simulink model "model_sim_CHBjt7"  (R2023b)
settings: Solver=ode3  StartTime=0.0  StopTime=5  FixedStep=01e-6  RelTol=1e-3
InitFcn:
  | sysinit
StopFcn:
  | code_CHBJT7_stopfcn
values from neighbouring files (symbols this model uses):
  C = 0.0234    [sysinit.m]
  f = 50    [sysinit.m]
  f_switch = 250    [sysinit.m]
  fn = 50    [sysinit.m]
  L = 0.002    [sysinit.m]
  L_1 = eps    [simout_chb_par.m]    (also in simout_chbjt_par.m; sysinit.m)
  L_ori = 0.02    [sysinit.m]
  L_sec = 0.06    [sysinit.m]
  m = 0.95    [sysinit.m]
  P0 = 8e6    (= 8000000)    [sysinit.m]
  R = 1.5    [sysinit.m]
  Source_Amp = 10000    [sysinit.m]
  st = 1e-6    (= 1e-06)    [sysinit.m]
  Td = 15e-7    (= 1.5e-06)    [sysinit.m]
  Ts2 = 0.5e-3    (= 0.0005)    [sysinit.m]
  U_dcN = 2500    [sysinit.m]
  Ul_in = 1900    [sysinit.m]
undefined symbols (not defined in the file or in its folder): magnitude
libraries: spsSeriesRLCBranchLib x120, spsDiodeLib x45, spsIGBTLib x36, spsMeanLib x20, spsCurrentMeasurementLib x15, spsThreePhaseVIMeasurementLib x10, spsOnDelayLib x9, spsMultiWindingTransformerLib x9, spsUniversalBridgeLib x9, simulink x5, spsVoltageMeasurementLib x5, spsRMSLib x4
(part 2 of 3)

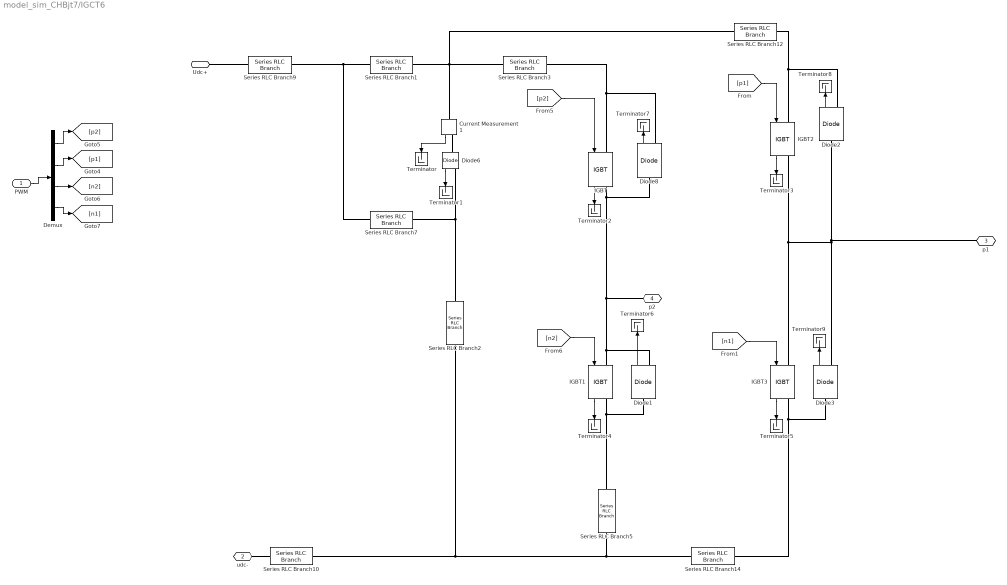
== system model_sim_CHBjt7/IGCT6 ==
  PWM : Inport
  Current Measurement1 : spsCurrentMeasurementLib/Current Measurement  PhasorSimulation=off  OutputType=Complex  PSBequivalent=0
  Demux : Demux
  Diode{1..3,6,8} (5 alike) : spsDiodeLib/Diode  Ron=rto  Lon=0  Vf=vto  IC=0  UseSnubber=off  Rs=500  Cs=250e-9  Measurements=on
  IGBT{,1..3} (4 alike) : spsIGBTLib/IGBT  Ron=rt  Lon=0  Vf=vt  Tf=1e-6  Tt=2e-6  IC=0  Rs=1e5  Cs=inf  Measurements=on
  Series RLC Branch1 : spsSeriesRLCBranchLib/Series RLC Branch  LConnTagsString=__new0  RConnTagsString=__new0  BranchType=RL  Resistance=1e-5  Inductance=3.0E-6  SetiL0=off  InitialCurrent=0  Capacitance=1e-6  Setx0=off  InitialVoltage=0  Measurements=None
  Series RLC Branch10 : spsSeriesRLCBranchLib/Series RLC Branch  LConnTagsString=__new0  RConnTagsString=__new0  BranchType=L  Resistance=1  Inductance=0.4e-6  SetiL0=off  InitialCurrent=0  Capacitance=1e-6  Setx0=off  InitialVoltage=0  Measurements=None
  Series RLC Branch12 : spsSeriesRLCBranchLib/Series RLC Branch  LConnTagsString=__new0  RConnTagsString=__new0  BranchType=RL  Resistance=1e-5  Inductance=1E-9  SetiL0=off  InitialCurrent=0  Capacitance=1e-6  Setx0=off  InitialVoltage=0  Measurements=None
  Series RLC Branch14 : spsSeriesRLCBranchLib/Series RLC Branch  LConnTagsString=__new0  RConnTagsString=__new0  BranchType=L  Resistance=1  Inductance=1E-7  SetiL0=off  InitialCurrent=0  Capacitance=1e-6  Setx0=off  InitialVoltage=0  Measurements=None
  Series RLC Branch2 : spsSeriesRLCBranchLib/Series RLC Branch  LConnTagsString=__new0  RConnTagsString=__new0  BranchType=RC  Resistance=1e-5  Inductance=20e-6  SetiL0=off  InitialCurrent=0  Capacitance=17e-6  Setx0=off  InitialVoltage=0  Measurements=None
  Series RLC Branch3 : spsSeriesRLCBranchLib/Series RLC Branch  LConnTagsString=__new0  RConnTagsString=__new0  BranchType=RL  Resistance=1e-5  Inductance=1E-9  SetiL0=off  InitialCurrent=0  Capacitance=1e-6  Setx0=off  InitialVoltage=0  Measurements=None
  Series RLC Branch5 : spsSeriesRLCBranchLib/Series RLC Branch  LConnTagsString=__new0  RConnTagsString=__new0  BranchType=L  Resistance=1  Inductance=1E-7  SetiL0=off  InitialCurrent=0  Capacitance=1e-6  Setx0=off  InitialVoltage=0  Measurements=None
  Series RLC Branch7 : spsSeriesRLCBranchLib/Series RLC Branch  LConnTagsString=__new0  RConnTagsString=__new0  BranchType=RL  Resistance=0.6  Inductance=1e-6  SetiL0=off  InitialCurrent=0  Capacitance=1e-6  Setx0=off  InitialVoltage=0  Measurements=None
  Series RLC Branch9 : spsSeriesRLCBranchLib/Series RLC Branch  LConnTagsString=__new0  RConnTagsString=__new0  BranchType=L  Resistance=1  Inductance=0.4e-6  SetiL0=off  InitialCurrent=0  Capacitance=1e-6  Setx0=off  InitialVoltage=0  Measurements=None
  Terminator{,1..9} (10 alike) : Terminator
  Udc+ : PMIOPort  Side=Left
  udc- : PMIOPort  Port=2  Side=Left
  p1 : PMIOPort  Port=3  Side=Right
  p2 : PMIOPort  Port=4  Side=Right
  wires:
  Diode3/1 -> Terminator9/1
  IGBT3/1 -> Terminator5/1
  [n1] -> IGBT3/1
  IGBT1/1 -> Terminator4/1
  IGBT2/1 -> Terminator3/1
  IGBT/1 -> Terminator2/1
  [n2] -> IGBT1/1
  [p1] -> IGBT2/1
  Current Measurement1/1 -> Terminator/1
  Diode2/1 -> Terminator8/1
  [p2] -> IGBT/1
  Diode8/1 -> Terminator7/1
  Diode1/1 -> Terminator6/1
  Diode6/1 -> Terminator1/1
  Demux/3 -> [n2]
  PWM/1 -> Demux/1
  Demux/1 -> [p2]
  Demux/2 -> [p1]
  Demux/4 -> [n1]
  connections:
  Series RLC Branch10/LConn1 -- udc-/RConn1
  Series RLC Branch9/LConn1 -- Udc+/RConn1
  Diode6/RConn1 -- Series RLC Branch7/RConn1 -- Series RLC Branch2/LConn1
  Current Measurement1/LConn1 -- Series RLC Branch1/RConn1 -- Series RLC Branch3/LConn1 -- Series RLC Branch12/LConn1
  Diode3/LConn1 -- IGBT3/RConn1 -- Series RLC Branch14/RConn1
  Series RLC Branch3/RConn1 -- IGBT/LConn1 -- Diode8/RConn1
  Diode1/LConn1 -- Series RLC Branch5/RConn1 -- IGBT1/RConn1
  Current Measurement1/RConn1 -- Diode6/LConn1
  Diode2/RConn1 -- Series RLC Branch12/RConn1 -- IGBT2/LConn1
  p1/RConn1 -- Diode2/LConn1 -- Diode3/RConn1 -- IGBT3/LConn1 -- IGBT2/RConn1
  Series RLC Branch5/LConn1 -- Series RLC Branch14/LConn1 -- Series RLC Branch10/RConn1 -- Series RLC Branch2/RConn1
  Series RLC Branch1/LConn1 -- Series RLC Branch7/LConn1 -- Series RLC Branch9/RConn1
  p2/RConn1 -- IGBT1/LConn1 -- Diode1/RConn1 -- Diode8/LConn1 -- IGBT/RConn1

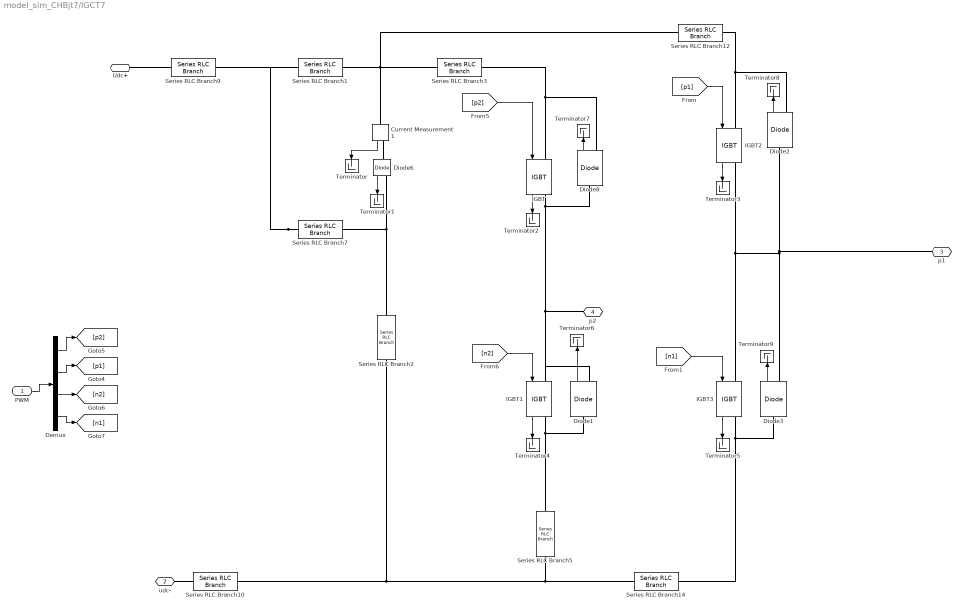
== system model_sim_CHBjt7/IGCT7 ==
  PWM : Inport
  Current Measurement1 : spsCurrentMeasurementLib/Current Measurement  PhasorSimulation=off  OutputType=Complex  PSBequivalent=0
  Demux : Demux
  Diode{1..3,6,8} (5 alike) : spsDiodeLib/Diode  Ron=rto  Lon=0  Vf=vto  IC=0  UseSnubber=off  Rs=500  Cs=250e-9  Measurements=on
  IGBT{,1..3} (4 alike) : spsIGBTLib/IGBT  Ron=rt  Lon=0  Vf=vt  Tf=1e-6  Tt=2e-6  IC=0  Rs=1e5  Cs=inf  Measurements=on
  Series RLC Branch1 : spsSeriesRLCBranchLib/Series RLC Branch  LConnTagsString=__new0  RConnTagsString=__new0  BranchType=RL  Resistance=1e-5  Inductance=3.0E-6  SetiL0=off  InitialCurrent=0  Capacitance=1e-6  Setx0=off  InitialVoltage=0  Measurements=None
  Series RLC Branch10 : spsSeriesRLCBranchLib/Series RLC Branch  LConnTagsString=__new0  RConnTagsString=__new0  BranchType=L  Resistance=1  Inductance=0.4e-6  SetiL0=off  InitialCurrent=0  Capacitance=1e-6  Setx0=off  InitialVoltage=0  Measurements=None
  Series RLC Branch12 : spsSeriesRLCBranchLib/Series RLC Branch  LConnTagsString=__new0  RConnTagsString=__new0  BranchType=RL  Resistance=1e-5  Inductance=1E-9  SetiL0=off  InitialCurrent=0  Capacitance=1e-6  Setx0=off  InitialVoltage=0  Measurements=None
  Series RLC Branch14 : spsSeriesRLCBranchLib/Series RLC Branch  LConnTagsString=__new0  RConnTagsString=__new0  BranchType=L  Resistance=1  Inductance=1E-7  SetiL0=off  InitialCurrent=0  Capacitance=1e-6  Setx0=off  InitialVoltage=0  Measurements=None
  Series RLC Branch2 : spsSeriesRLCBranchLib/Series RLC Branch  LConnTagsString=__new0  RConnTagsString=__new0  BranchType=RC  Resistance=1e-5  Inductance=20e-6  SetiL0=off  InitialCurrent=0  Capacitance=17e-6  Setx0=off  InitialVoltage=0  Measurements=None
  Series RLC Branch3 : spsSeriesRLCBranchLib/Series RLC Branch  LConnTagsString=__new0  RConnTagsString=__new0  BranchType=RL  Resistance=1e-5  Inductance=1E-9  SetiL0=off  InitialCurrent=0  Capacitance=1e-6  Setx0=off  InitialVoltage=0  Measurements=None
  Series RLC Branch5 : spsSeriesRLCBranchLib/Series RLC Branch  LConnTagsString=__new0  RConnTagsString=__new0  BranchType=L  Resistance=1  Inductance=1E-7  SetiL0=off  InitialCurrent=0  Capacitance=1e-6  Setx0=off  InitialVoltage=0  Measurements=None
  Series RLC Branch7 : spsSeriesRLCBranchLib/Series RLC Branch  LConnTagsString=__new0  RConnTagsString=__new0  BranchType=RL  Resistance=0.6  Inductance=1e-6  SetiL0=off  InitialCurrent=0  Capacitance=1e-6  Setx0=off  InitialVoltage=0  Measurements=None
  Series RLC Branch9 : spsSeriesRLCBranchLib/Series RLC Branch  LConnTagsString=__new0  RConnTagsString=__new0  BranchType=L  Resistance=1  Inductance=0.4e-6  SetiL0=off  InitialCurrent=0  Capacitance=1e-6  Setx0=off  InitialVoltage=0  Measurements=None
  Terminator{,1..9} (10 alike) : Terminator
  Udc+ : PMIOPort  Side=Left
  udc- : PMIOPort  Port=2  Side=Left
  p1 : PMIOPort  Port=3  Side=Right
  p2 : PMIOPort  Port=4  Side=Right
  wires:
  Diode6/1 -> Terminator1/1
  Diode1/1 -> Terminator6/1
  Diode8/1 -> Terminator7/1
  PWM/1 -> Demux/1
  [p2] -> IGBT/1
  Diode2/1 -> Terminator8/1
  Current Measurement1/1 -> Terminator/1
  [p1] -> IGBT2/1
  [n2] -> IGBT1/1
  IGBT/1 -> Terminator2/1
  IGBT2/1 -> Terminator3/1
  Demux/4 -> [n1]
  Demux/3 -> [n2]
  Demux/2 -> [p1]
  IGBT1/1 -> Terminator4/1
  [n1] -> IGBT3/1
  IGBT3/1 -> Terminator5/1
  Diode3/1 -> Terminator9/1
  Demux/1 -> [p2]
  connections:
  IGBT/RConn1 -- Diode8/LConn1 -- p2/RConn1 -- Diode1/RConn1 -- IGBT1/LConn1
  Series RLC Branch7/LConn1 -- Series RLC Branch1/LConn1 -- Series RLC Branch9/RConn1
  Series RLC Branch14/LConn1 -- Series RLC Branch2/RConn1 -- Series RLC Branch10/RConn1 -- Series RLC Branch5/LConn1
  Diode2/LConn1 -- IGBT2/RConn1 -- IGBT3/LConn1 -- Diode3/RConn1 -- p1/RConn1
  Series RLC Branch12/RConn1 -- IGBT2/LConn1 -- Diode2/RConn1
  Current Measurement1/RConn1 -- Diode6/LConn1
  Series RLC Branch5/RConn1 -- Diode1/LConn1 -- IGBT1/RConn1
  IGBT/LConn1 -- Diode8/RConn1 -- Series RLC Branch3/RConn1
  IGBT3/RConn1 -- Diode3/LConn1 -- Series RLC Branch14/RConn1
  Series RLC Branch1/RConn1 -- Current Measurement1/LConn1 -- Series RLC Branch12/LConn1 -- Series RLC Branch3/LConn1
  Series RLC Branch7/RConn1 -- Diode6/RConn1 -- Series RLC Branch2/LConn1
  Series RLC Branch9/LConn1 -- Udc+/RConn1
  Series RLC Branch10/LConn1 -- udc-/RConn1

== system model_sim_CHBjt7/IGCT8 ==
  PWM : Inport
  Current Measurement1 : spsCurrentMeasurementLib/Current Measurement  PhasorSimulation=off  OutputType=Complex  PSBequivalent=0
  Demux : Demux
  Diode{1..3,6,8} (5 alike) : spsDiodeLib/Diode  Ron=rto  Lon=0  Vf=vto  IC=0  UseSnubber=off  Rs=500  Cs=250e-9  Measurements=on
  IGBT{,1..3} (4 alike) : spsIGBTLib/IGBT  Ron=rt  Lon=0  Vf=vt  Tf=1e-6  Tt=2e-6  IC=0  Rs=1e5  Cs=inf  Measurements=on
  Series RLC Branch1 : spsSeriesRLCBranchLib/Series RLC Branch  LConnTagsString=__new0  RConnTagsString=__new0  BranchType=RL  Resistance=1e-5  Inductance=3.0E-6  SetiL0=off  InitialCurrent=0  Capacitance=1e-6  Setx0=off  InitialVoltage=0  Measurements=None
  Series RLC Branch10 : spsSeriesRLCBranchLib/Series RLC Branch  LConnTagsString=__new0  RConnTagsString=__new0  BranchType=L  Resistance=1  Inductance=0.4e-6  SetiL0=off  InitialCurrent=0  Capacitance=1e-6  Setx0=off  InitialVoltage=0  Measurements=None
  Series RLC Branch12 : spsSeriesRLCBranchLib/Series RLC Branch  LConnTagsString=__new0  RConnTagsString=__new0  BranchType=RL  Resistance=1e-5  Inductance=1E-9  SetiL0=off  InitialCurrent=0  Capacitance=1e-6  Setx0=off  InitialVoltage=0  Measurements=None
  Series RLC Branch14 : spsSeriesRLCBranchLib/Series RLC Branch  LConnTagsString=__new0  RConnTagsString=__new0  BranchType=L  Resistance=1  Inductance=1E-7  SetiL0=off  InitialCurrent=0  Capacitance=1e-6  Setx0=off  InitialVoltage=0  Measurements=None
  Series RLC Branch2 : spsSeriesRLCBranchLib/Series RLC Branch  LConnTagsString=__new0  RConnTagsString=__new0  BranchType=RC  Resistance=1e-5  Inductance=20e-6  SetiL0=off  InitialCurrent=0  Capacitance=17e-6  Setx0=off  InitialVoltage=0  Measurements=None
  Series RLC Branch3 : spsSeriesRLCBranchLib/Series RLC Branch  LConnTagsString=__new0  RConnTagsString=__new0  BranchType=RL  Resistance=1e-5  Inductance=1E-9  SetiL0=off  InitialCurrent=0  Capacitance=1e-6  Setx0=off  InitialVoltage=0  Measurements=None
  Series RLC Branch5 : spsSeriesRLCBranchLib/Series RLC Branch  LConnTagsString=__new0  RConnTagsString=__new0  BranchType=L  Resistance=1  Inductance=1E-7  SetiL0=off  InitialCurrent=0  Capacitance=1e-6  Setx0=off  InitialVoltage=0  Measurements=None
  Series RLC Branch7 : spsSeriesRLCBranchLib/Series RLC Branch  LConnTagsString=__new0  RConnTagsString=__new0  BranchType=RL  Resistance=0.6  Inductance=1e-6  SetiL0=off  InitialCurrent=0  Capacitance=1e-6  Setx0=off  InitialVoltage=0  Measurements=None
  Series RLC Branch9 : spsSeriesRLCBranchLib/Series RLC Branch  LConnTagsString=__new0  RConnTagsString=__new0  BranchType=L  Resistance=1  Inductance=0.4e-6  SetiL0=off  InitialCurrent=0  Capacitance=1e-6  Setx0=off  InitialVoltage=0  Measurements=None
  Terminator{,1..9} (10 alike) : Terminator
  Udc+ : PMIOPort  Side=Left
  udc- : PMIOPort  Port=2  Side=Left
  p1 : PMIOPort  Port=3  Side=Right
  p2 : PMIOPort  Port=4  Side=Right
  wires:
  Diode3/1 -> Terminator9/1
  IGBT3/1 -> Terminator5/1
  [n1] -> IGBT3/1
  IGBT1/1 -> Terminator4/1
  IGBT2/1 -> Terminator3/1
  IGBT/1 -> Terminator2/1
  [n2] -> IGBT1/1
  [p1] -> IGBT2/1
  Current Measurement1/1 -> Terminator/1
  Diode2/1 -> Terminator8/1
  [p2] -> IGBT/1
  Diode8/1 -> Terminator7/1
  Diode1/1 -> Terminator6/1
  Diode6/1 -> Terminator1/1
  Demux/3 -> [n2]
  PWM/1 -> Demux/1
  Demux/1 -> [p2]
  Demux/2 -> [p1]
  Demux/4 -> [n1]
  connections:
  Series RLC Branch10/LConn1 -- udc-/RConn1
  Series RLC Branch9/LConn1 -- Udc+/RConn1
  Diode6/RConn1 -- Series RLC Branch7/RConn1 -- Series RLC Branch2/LConn1
  Current Measurement1/LConn1 -- Series RLC Branch1/RConn1 -- Series RLC Branch3/LConn1 -- Series RLC Branch12/LConn1
  Diode3/LConn1 -- IGBT3/RConn1 -- Series RLC Branch14/RConn1
  Series RLC Branch3/RConn1 -- IGBT/LConn1 -- Diode8/RConn1
  Diode1/LConn1 -- Series RLC Branch5/RConn1 -- IGBT1/RConn1
  Current Measurement1/RConn1 -- Diode6/LConn1
  Diode2/RConn1 -- Series RLC Branch12/RConn1 -- IGBT2/LConn1
  p1/RConn1 -- Diode2/LConn1 -- Diode3/RConn1 -- IGBT3/LConn1 -- IGBT2/RConn1
  Series RLC Branch5/LConn1 -- Series RLC Branch14/LConn1 -- Series RLC Branch10/RConn1 -- Series RLC Branch2/RConn1
  Series RLC Branch1/LConn1 -- Series RLC Branch7/LConn1 -- Series RLC Branch9/RConn1
  p2/RConn1 -- IGBT1/LConn1 -- Diode1/RConn1 -- Diode8/LConn1 -- IGBT/RConn1

== system model_sim_CHBjt7/IGCT9 ==
  PWM : Inport
  Current Measurement1 : spsCurrentMeasurementLib/Current Measurement  PhasorSimulation=off  OutputType=Complex  PSBequivalent=0
  Demux : Demux
  Diode{1..3,6,8} (5 alike) : spsDiodeLib/Diode  Ron=rto  Lon=0  Vf=vto  IC=0  UseSnubber=off  Rs=500  Cs=250e-9  Measurements=on
  IGBT{,1..3} (4 alike) : spsIGBTLib/IGBT  Ron=rt  Lon=0  Vf=vt  Tf=1e-6  Tt=2e-6  IC=0  Rs=1e5  Cs=inf  Measurements=on
  Series RLC Branch1 : spsSeriesRLCBranchLib/Series RLC Branch  LConnTagsString=__new0  RConnTagsString=__new0  BranchType=RL  Resistance=1e-5  Inductance=3.0E-6  SetiL0=off  InitialCurrent=0  Capacitance=1e-6  Setx0=off  InitialVoltage=0  Measurements=None
  Series RLC Branch10 : spsSeriesRLCBranchLib/Series RLC Branch  LConnTagsString=__new0  RConnTagsString=__new0  BranchType=L  Resistance=1  Inductance=0.4e-6  SetiL0=off  InitialCurrent=0  Capacitance=1e-6  Setx0=off  InitialVoltage=0  Measurements=None
  Series RLC Branch12 : spsSeriesRLCBranchLib/Series RLC Branch  LConnTagsString=__new0  RConnTagsString=__new0  BranchType=RL  Resistance=1e-5  Inductance=1E-9  SetiL0=off  InitialCurrent=0  Capacitance=1e-6  Setx0=off  InitialVoltage=0  Measurements=None
  Series RLC Branch14 : spsSeriesRLCBranchLib/Series RLC Branch  LConnTagsString=__new0  RConnTagsString=__new0  BranchType=L  Resistance=1  Inductance=1E-7  SetiL0=off  InitialCurrent=0  Capacitance=1e-6  Setx0=off  InitialVoltage=0  Measurements=None
  Series RLC Branch2 : spsSeriesRLCBranchLib/Series RLC Branch  LConnTagsString=__new0  RConnTagsString=__new0  BranchType=RC  Resistance=1e-5  Inductance=20e-6  SetiL0=off  InitialCurrent=0  Capacitance=17e-6  Setx0=off  InitialVoltage=0  Measurements=None
  Series RLC Branch3 : spsSeriesRLCBranchLib/Series RLC Branch  LConnTagsString=__new0  RConnTagsString=__new0  BranchType=RL  Resistance=1e-5  Inductance=1E-9  SetiL0=off  InitialCurrent=0  Capacitance=1e-6  Setx0=off  InitialVoltage=0  Measurements=None
  Series RLC Branch5 : spsSeriesRLCBranchLib/Series RLC Branch  LConnTagsString=__new0  RConnTagsString=__new0  BranchType=L  Resistance=1  Inductance=1E-7  SetiL0=off  InitialCurrent=0  Capacitance=1e-6  Setx0=off  InitialVoltage=0  Measurements=None
  Series RLC Branch7 : spsSeriesRLCBranchLib/Series RLC Branch  LConnTagsString=__new0  RConnTagsString=__new0  BranchType=RL  Resistance=0.6  Inductance=1e-6  SetiL0=off  InitialCurrent=0  Capacitance=1e-6  Setx0=off  InitialVoltage=0  Measurements=None
  Series RLC Branch9 : spsSeriesRLCBranchLib/Series RLC Branch  LConnTagsString=__new0  RConnTagsString=__new0  BranchType=L  Resistance=1  Inductance=0.4e-6  SetiL0=off  InitialCurrent=0  Capacitance=1e-6  Setx0=off  InitialVoltage=0  Measurements=None
  Terminator{,1..9} (10 alike) : Terminator
  Udc+ : PMIOPort  Side=Left
  udc- : PMIOPort  Port=2  Side=Left
  p1 : PMIOPort  Port=3  Side=Right
  p2 : PMIOPort  Port=4  Side=Right
  wires:
  Diode3/1 -> Terminator9/1
  IGBT3/1 -> Terminator5/1
  [n1] -> IGBT3/1
  IGBT1/1 -> Terminator4/1
  IGBT2/1 -> Terminator3/1
  IGBT/1 -> Terminator2/1
  [n2] -> IGBT1/1
  [p1] -> IGBT2/1
  Current Measurement1/1 -> Terminator/1
  Diode2/1 -> Terminator8/1
  [p2] -> IGBT/1
  Diode8/1 -> Terminator7/1
  Diode1/1 -> Terminator6/1
  Diode6/1 -> Terminator1/1
  Demux/3 -> [n2]
  PWM/1 -> Demux/1
  Demux/1 -> [p2]
  Demux/2 -> [p1]
  Demux/4 -> [n1]
  connections:
  Series RLC Branch10/LConn1 -- udc-/RConn1
  Series RLC Branch9/LConn1 -- Udc+/RConn1
  Diode6/RConn1 -- Series RLC Branch7/RConn1 -- Series RLC Branch2/LConn1
  Current Measurement1/LConn1 -- Series RLC Branch1/RConn1 -- Series RLC Branch3/LConn1 -- Series RLC Branch12/LConn1
  Diode3/LConn1 -- IGBT3/RConn1 -- Series RLC Branch14/RConn1
  Series RLC Branch3/RConn1 -- IGBT/LConn1 -- Diode8/RConn1
  Diode1/LConn1 -- Series RLC Branch5/RConn1 -- IGBT1/RConn1
  Current Measurement1/RConn1 -- Diode6/LConn1
  Diode2/RConn1 -- Series RLC Branch12/RConn1 -- IGBT2/LConn1
  p1/RConn1 -- Diode2/LConn1 -- Diode3/RConn1 -- IGBT3/LConn1 -- IGBT2/RConn1
  Series RLC Branch5/LConn1 -- Series RLC Branch14/LConn1 -- Series RLC Branch10/RConn1 -- Series RLC Branch2/RConn1
  Series RLC Branch1/LConn1 -- Series RLC Branch7/LConn1 -- Series RLC Branch9/RConn1
  p2/RConn1 -- IGBT1/LConn1 -- Diode1/RConn1 -- Diode8/LConn1 -- IGBT/RConn1

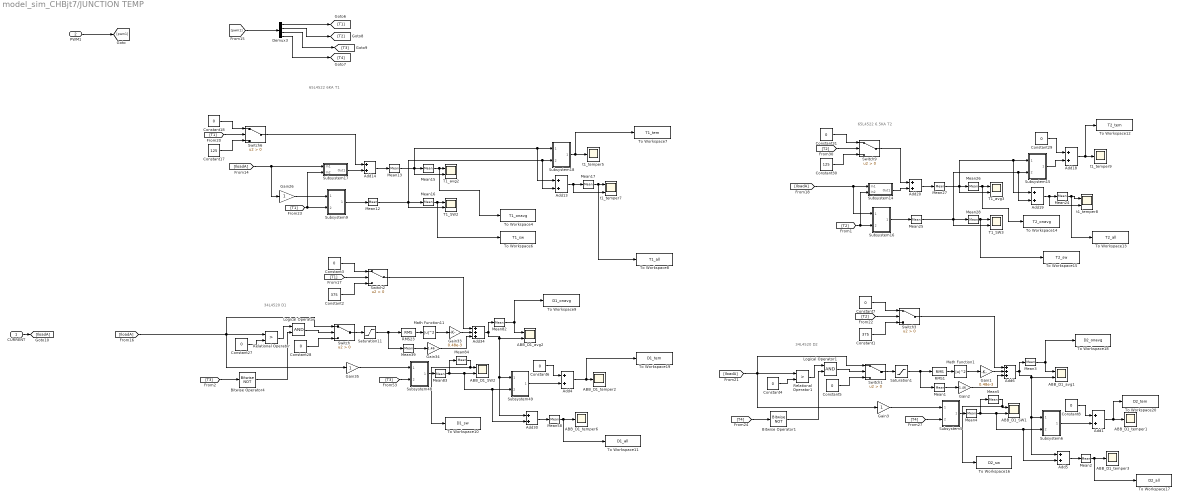
== system model_sim_CHBjt7/JUNCTION TEMP ==
  note: 65L4522 6.5KA T2
  note: 34L4520 D1
  note: 34L4520 D2
  note: 65L4522 6KA T1
  CURRENT : Inport
  PWM1 : Inport  Port=2
  ABB_D1_SW1 : Scope  NumInputPorts=2
  ABB_D1_SW2 : Scope  NumInputPorts=2
  ABB_D1_avg1 : Scope  NumInputPorts=2
  ABB_D1_avg2 : Scope  NumInputPorts=2
  ABB_D1_temper{1..3,6} (4 alike) : Scope
  Add{1,4..5,13..14,18..20,30} (9 alike) : Sum
  Add34 : Sum  Inputs=+++
  Add6 : Sum  Inputs=+++
  Bitwise Operator1 : simulink/Logic and Bit Operations/Bitwise Operator  logicop=NOT  UseBitMask=off  BitMask=bin2dec('11011001')  BitMaskRealWorld=Stored Integer
  Bitwise Operator4 : simulink/Logic and Bit Operations/Bitwise Operator  logicop=NOT  UseBitMask=off  BitMask=bin2dec('11011001')  BitMaskRealWorld=Stored Integer
  Constant1 : Constant  Value=375
  Constant17 : Constant  Value=125
  Constant{3..8,18,27..29,31} (11 alike) : Constant  Value=0
  Constant2 : Constant  Value=375
  Constant30 : Constant  Value=125
  Demux3 : Demux
  Gain1 : Gain  Gain=0.48e-3
  Gain2 : Gain  Gain=1.46
  Gain26 : Gain
  Gain3 : Gain
  Gain33 : Gain  Gain=0.48e-3
  Gain34 : Gain  Gain=1.46
  Gain35 : Gain
  Logical Operator : Logic  AllPortsSameDT=off  OutDataTypeStr=boolean
  Logical Operator1 : Logic  AllPortsSameDT=off  OutDataTypeStr=boolean
  Math Function1 : Math  Operator=magnitude^2  SignedPower=on
  Math Function11 : Math  Operator=magnitude^2  SignedPower=on
  Mean{1,4,12..13,25,27,39,83} (8 alike) : spsMeanLib/Mean  Freq=2000  Vinit=0  Ts=1e-6
  Mean{15..16,26,28} (4 alike) : spsMeanLib/Mean  Freq=f  Vinit=0  Ts=Ts2
  Mean{2..3,5,17,24,58,82,84} (8 alike) : spsMeanLib/Mean  Freq=f  Vinit=0  Ts=1e-6
  RMS1 : spsRMSLib/RMS  TrueRMS=on  Freq=2000  RMSInit=0  Ts=1e-6
  RMS23 : spsRMSLib/RMS  TrueRMS=on  Freq=2000  RMSInit=0  Ts=1e-6
  Relational Operator : RelationalOperator  Operator=>  OutDataTypeStr=boolean  RndMeth=Simplest  InputSameDT=off
  Relational Operator1 : RelationalOperator  Operator=>  OutDataTypeStr=boolean  RndMeth=Simplest  InputSameDT=off
  Saturation1 : Saturate  UpperLimit=5500  LowerLimit=0
  Saturation11 : Saturate  UpperLimit=5500  LowerLimit=0
  Subsystem14 : Subsystem
  Subsystem15 : Subsystem
  Subsystem16 : Subsystem
  Subsystem17 : Subsystem
  Subsystem18 : Subsystem
  Subsystem48 : Subsystem
  Subsystem49 : Subsystem
  Subsystem5 : Subsystem
  Subsystem6 : Subsystem
  Subsystem9 : Subsystem
  Switch{,1..3,6,9} (6 alike) : Switch  Criteria=u2 > Threshold  SaturateOnIntegerOverflow=off  InputSameDT=off
  T1_SW2 : Scope  NumInputPorts=2
  T1_SW3 : Scope  NumInputPorts=2
  T1_avg2 : Scope  NumInputPorts=2
  T1_avg3 : Scope  NumInputPorts=2
  To Workspace10 : ToWorkspace  VariableName=D1_sw  SaveFormat=Structure With Time  SampleTime=-1
  To Workspace11 : ToWorkspace  VariableName=D1_all  SaveFormat=Structure With Time  SampleTime=-1
  To Workspace12 : ToWorkspace  VariableName=T2_tem  SaveFormat=Structure With Time  SampleTime=-1
  To Workspace13 : ToWorkspace  VariableName=T2_all  SaveFormat=Structure With Time  SampleTime=-1
  To Workspace14 : ToWorkspace  VariableName=T2_onavg  SaveFormat=Structure With Time  SampleTime=-1
  To Workspace15 : ToWorkspace  VariableName=T2_sw  SaveFormat=Structure With Time  SampleTime=-1
  To Workspace16 : ToWorkspace  VariableName=D2_sw  SaveFormat=Structure With Time  SampleTime=-1
  To Workspace17 : ToWorkspace  VariableName=D2_all  SaveFormat=Structure With Time  SampleTime=-1
  To Workspace18 : ToWorkspace  VariableName=D2_onavg  SaveFormat=Structure With Time  SampleTime=-1
  To Workspace19 : ToWorkspace  VariableName=D1_tem  SaveFormat=Structure With Time  SampleTime=-1
  To Workspace20 : ToWorkspace  VariableName=D2_tem  SaveFormat=Structure With Time  SampleTime=-1
  To Workspace4 : ToWorkspace  VariableName=T1_onavg  SaveFormat=Structure With Time  SampleTime=-1
  To Workspace6 : ToWorkspace  VariableName=T1_sw  SaveFormat=Structure With Time  SampleTime=-1
  To Workspace7 : ToWorkspace  VariableName=T1_tem  SaveFormat=Structure With Time  SampleTime=-1
  To Workspace8 : ToWorkspace  VariableName=T1_all  SaveFormat=Structure With Time  SampleTime=-1
  To Workspace9 : ToWorkspace  VariableName=D1_onavg  SaveFormat=Structure With Time  SampleTime=-1
  t1_temper5 : Scope
  t1_temper7 : Scope  NumInputPorts=2
  t1_temper8 : Scope  NumInputPorts=2
  t1_temper9 : Scope
  wires:
  Mean24/1 -> To Workspace13/1, t1_temper8/1
  Mean13/1 -> T1_avg2/2, Mean15/1, Subsystem18/1(In1), Add13/1
  Add1/1 -> To Workspace20/1, ABB_D1_temper1/1
  Add20/1 -> Mean27/1
  Constant18/1 -> Switch6/1
  [T2] -> Switch9/2
  RMS1/1 -> Math Function1/1
  [T1] -> Subsystem9/2(In2), Subsystem17/2(In2)
  Saturation1/1 -> RMS1/1, Mean1/1
  Mean17/1 -> To Workspace8/1, t1_temper7/1
  Demux3/2 -> [T2]
  Mean12/1 -> Subsystem18/2(In2), Add13/2, T1_SW2/2, Mean16/1
  Bitwise Operator1/1 -> Logical Operator1/2
  Add5/1 -> Mean2/1
  Mean84/1 -> To Workspace10/1, ABB_D1_SW2/1
  Demux3/3 -> [T3]
  RMS23/1 -> Math Function11/1
  Add6/1 -> Mean3/1, ABB_D1_avg1/2, Subsystem6/1(In1), Add5/1
  Mean3/1 -> To Workspace18/1, ABB_D1_avg1/1
  [T3] -> Subsystem48/2(In2)
  Mean58/1 -> ABB_D1_temper6/1, To Workspace11/1
  Bitwise Operator4/1 -> Logical Operator/2
  Logical Operator/1 -> Switch/2
  Constant8/1 -> Add1/1
  Add14/1 -> Mean13/1
  Subsystem6/1(Out1) -> Add1/2
  Mean27/1 -> T1_avg3/2, Mean26/1, Subsystem15/1(In1), Add19/1
  Gain35/1 -> Subsystem48/1(In1)
  Add34/1 -> Add30/1, Subsystem49/1(In1), ABB_D1_avg2/2, Mean82/1
  Constant3/1 -> Switch2/1
  Math Function1/1 -> Gain1/1
  Subsystem18/1(Out1) -> To Workspace7/1, t1_temper5/1
  Subsystem5/1(Out1) -> Mean4/1
  Mean5/1 -> ABB_D1_SW1/1, To Workspace16/1
  Constant27/1 -> Relational Operator/2
  Switch9/1 -> Add20/1
  Gain3/1 -> Subsystem5/1(In1)
  Switch6/1 -> Add14/1
  Constant5/1 -> Switch1/3
  Constant6/1 -> Add4/1
  Relational Operator1/1 -> Logical Operator1/1
  Constant1/1 -> Switch3/3
  [pwm1] -> Demux3/1
  Gain34/1 -> Add34/3
  Constant7/1 -> Switch3/1
  [T4] -> Subsystem5/2(In2)
  [IloadA] -> Subsystem16/1(In1), Subsystem14/1(In1)
  Constant4/1 -> Relational Operator1/2
  [T2] -> Switch3/2
  Switch/1 -> Saturation11/1
  Demux3/1 -> [T1]
  Mean28/1 -> To Workspace15/1, T1_SW3/1
  Add19/1 -> t1_temper8/2, Mean24/1
  [IloadA] -> Relational Operator1/1, Gain3/1, Switch1/1
  Add4/1 -> To Workspace19/1, ABB_D1_temper2/1
  Add18/1 -> To Workspace12/1, t1_temper9/1
  [IloadA] -> Gain26/1, Subsystem17/1(In1)
  Demux3/4 -> [T4]
  Subsystem14/1(Out1) -> Add20/2
  Gain1/1 -> Add6/2
  Subsystem9/1(Out1) -> Mean12/1
  Switch1/1 -> Saturation1/1
  Logical Operator1/1 -> Switch1/2
  Subsystem16/1(Out1) -> Mean25/1
  Subsystem17/1(Out1) -> Add14/2
  Relational Operator/1 -> Logical Operator/1
  [T2] -> Subsystem14/2(In2), Subsystem16/2(In2)
  Gain2/1 -> Add6/3
  Constant2/1 -> Switch2/3
  Constant31/1 -> Switch9/1
  Constant29/1 -> Add18/1
  Mean82/1 -> ABB_D1_avg2/1, To Workspace9/1
  [T1] -> Switch2/2
  Gain26/1 -> Subsystem9/1(In1)
  Constant30/1 -> Switch9/3
  Subsystem15/1(Out1) -> Add18/2
  Mean83/1 -> Mean84/1, Add30/2, Subsystem49/2(In2), ABB_D1_SW2/2
  Mean25/1 -> Subsystem15/2(In2), Add19/2, T1_SW3/2, Mean28/1
  Mean26/1 -> To Workspace14/1, T1_avg3/1
  Subsystem48/1(Out1) -> Mean83/1
  Constant28/1 -> Switch/3
  Math Function11/1 -> Gain33/1
  Switch2/1 -> Add34/1
  Switch3/1 -> Add6/1
  Mean4/1 -> ABB_D1_SW1/2, Subsystem6/2(In2), Add5/2, Mean5/1
  [T3] -> Bitwise Operator4/1
  Mean16/1 -> To Workspace6/1, T1_SW2/1
  Saturation11/1 -> Mean39/1, RMS23/1
  Mean15/1 -> To Workspace4/1, T1_avg2/1
  [IloadA] -> Switch/1, Gain35/1, Relational Operator/1
  Add30/1 -> Mean58/1
  Mean2/1 -> To Workspace17/1, ABB_D1_temper3/1
  Add13/1 -> t1_temper7/2, Mean17/1
  [T4] -> Bitwise Operator1/1
  Subsystem49/1(Out1) -> Add4/2
  Constant17/1 -> Switch6/3
  Gain33/1 -> Add34/2
  Mean39/1 -> Gain34/1
  Mean1/1 -> Gain2/1
  [T1] -> Switch6/2
  CURRENT/1 -> [IloadA]
  PWM1/1 -> [pwm1]

== system model_sim_CHBjt7/LOAD ==
  Series RLC Branch1 : spsSeriesRLCBranchLib/Series RLC Branch  LConnTagsString=__new0  RConnTagsString=__new0  BranchType=RL  Resistance=R*1.5  Inductance=L*1.5  SetiL0=off  InitialCurrent=0  Capacitance=1e-6  Setx0=off  InitialVoltage=0  Measurements=None
  Series RLC Branch2 : spsSeriesRLCBranchLib/Series RLC Branch  LConnTagsString=__new0  RConnTagsString=__new0  BranchType=RL  Resistance=R*1.5  Inductance=L*1.5  SetiL0=off  InitialCurrent=0  Capacitance=1e-6  Setx0=off  InitialVoltage=0  Measurements=None
  Series RLC Branch7 : spsSeriesRLCBranchLib/Series RLC Branch  LConnTagsString=__new0  RConnTagsString=__new0  BranchType=RL  Resistance=R*1.5  Inductance=L*1.5  SetiL0=off  InitialCurrent=0  Capacitance=1e-6  Setx0=off  InitialVoltage=0  Measurements=None
  A : PMIOPort  Side=Left
  B : PMIOPort  Port=2  Side=Left
  C : PMIOPort  Port=3  Side=Left
  connections:
  Series RLC Branch7/RConn1 -- Series RLC Branch2/RConn1 -- Series RLC Branch1/RConn1
  Series RLC Branch2/LConn1 -- C/RConn1
  Series RLC Branch7/LConn1 -- A/RConn1
  Series RLC Branch1/LConn1 -- B/RConn1

== system model_sim_CHBjt7/Subsystem ==
  Current Measurement : spsCurrentMeasurementLib/Current Measurement  PhasorSimulation=off  OutputType=Complex  PSBequivalent=0
  Voltage Measurement : spsVoltageMeasurementLib/Voltage Measurement  PhasorSimulation=off  OutputType=Complex  PSBequivalent=0
  + : PMIOPort  Side=Left
  - : PMIOPort  Port=2  Side=Left
  +OUT : PMIOPort  Port=3  Side=Right
  -OUT : PMIOPort  Port=4  Side=Right
  tag scope: Idc1=global, Udc=global
  wires:
  Voltage Measurement/1 -> [Udc]
  Current Measurement/1 -> [Idc1]
  connections:
  Voltage Measurement/LConn1 -- Current Measurement/LConn1 -- +/RConn1
  Voltage Measurement/LConn2 -- -OUT/RConn1 -- -/RConn1
  Current Measurement/RConn1 -- +OUT/RConn1

== system model_sim_CHBjt7/Subsystem1 ==
  Current Measurement : spsCurrentMeasurementLib/Current Measurement  PhasorSimulation=off  OutputType=Complex  PSBequivalent=0
  Voltage Measurement : spsVoltageMeasurementLib/Voltage Measurement  PhasorSimulation=off  OutputType=Complex  PSBequivalent=0
  + : PMIOPort  Side=Left
  - : PMIOPort  Port=2  Side=Left
  +OUT : PMIOPort  Port=3  Side=Right
  -OUT : PMIOPort  Port=4  Side=Right
  tag scope: Idc2=global
  wires:
  Current Measurement/1 -> [Idc2]
  connections:
  Voltage Measurement/LConn1 -- +/RConn1 -- Current Measurement/LConn1
  Voltage Measurement/LConn2 -- -OUT/RConn1 -- -/RConn1
  Current Measurement/RConn1 -- +OUT/RConn1

== system model_sim_CHBjt7/Subsystem2 ==
  Current Measurement : spsCurrentMeasurementLib/Current Measurement  PhasorSimulation=off  OutputType=Complex  PSBequivalent=0
  Voltage Measurement : spsVoltageMeasurementLib/Voltage Measurement  PhasorSimulation=off  OutputType=Complex  PSBequivalent=0
  + : PMIOPort  Side=Left
  - : PMIOPort  Port=2  Side=Left
  +OUT : PMIOPort  Port=3  Side=Right
  -OUT : PMIOPort  Port=4  Side=Right
  tag scope: Idc3=global
  wires:
  Current Measurement/1 -> [Idc3]
  connections:
  Voltage Measurement/LConn1 -- +/RConn1 -- Current Measurement/LConn1
  Voltage Measurement/LConn2 -- -OUT/RConn1 -- -/RConn1
  Current Measurement/RConn1 -- +OUT/RConn1

== system model_sim_CHBjt7/Subsystem3 ==
  Series RLC Branch{1..9} (9 alike) : spsSeriesRLCBranchLib/Series RLC Branch  LConnTagsString=__new0  RConnTagsString=__new0  BranchType=L  Resistance=R*1.5  Inductance=L_in  SetiL0=off  InitialCurrent=0  Capacitance=1e-6  Setx0=off  InitialVoltage=0  Measurements=None
  Conn1 : PMIOPort  Side=Left
  Conn2 : PMIOPort  Port=2  Side=Right
  Conn3 : PMIOPort  Port=3  Side=Left
  Conn4 : PMIOPort  Port=4  Side=Right
  Conn5 : PMIOPort  Port=5  Side=Left
  Conn6 : PMIOPort  Port=6  Side=Right
  Conn7 : PMIOPort  Port=7  Side=Left
  Conn8 : PMIOPort  Port=8  Side=Right
  Conn9 : PMIOPort  Port=9  Side=Left
  Conn10 : PMIOPort  Port=10  Side=Right
  Conn11 : PMIOPort  Port=11  Side=Left
  Conn12 : PMIOPort  Port=12  Side=Right
  Conn13 : PMIOPort  Port=13  Side=Left
  Conn14 : PMIOPort  Port=14  Side=Right
  Conn15 : PMIOPort  Port=15  Side=Left
  Conn16 : PMIOPort  Port=16  Side=Right
  Conn17 : PMIOPort  Port=17  Side=Left
  Conn18 : PMIOPort  Port=18  Side=Right
  connections:
  Series RLC Branch3/RConn1 -- Conn8/RConn1
  Series RLC Branch3/LConn1 -- Conn7/RConn1
  Series RLC Branch7/LConn1 -- Conn1/RConn1
  Series RLC Branch7/RConn1 -- Conn2/RConn1
  Series RLC Branch1/LConn1 -- Conn3/RConn1
  Series RLC Branch2/LConn1 -- Conn5/RConn1
  Series RLC Branch4/LConn1 -- Conn9/RConn1
  Series RLC Branch5/LConn1 -- Conn11/RConn1
  Series RLC Branch4/RConn1 -- Conn10/RConn1
  Series RLC Branch1/RConn1 -- Conn4/RConn1
  Series RLC Branch5/RConn1 -- Conn12/RConn1
  Series RLC Branch9/LConn1 -- Conn17/RConn1
  Series RLC Branch8/LConn1 -- Conn15/RConn1
  Series RLC Branch6/RConn1 -- Conn14/RConn1
  Series RLC Branch9/RConn1 -- Conn18/RConn1
  Series RLC Branch8/RConn1 -- Conn16/RConn1
  Series RLC Branch6/LConn1 -- Conn13/RConn1
  Series RLC Branch2/RConn1 -- Conn6/RConn1

== system model_sim_CHBjt7/Subsystem4 ==
  Series RLC Branch{1..9} (9 alike) : spsSeriesRLCBranchLib/Series RLC Branch  LConnTagsString=__new0  RConnTagsString=__new0  BranchType=L  Resistance=R*1.5  Inductance=L_in  SetiL0=off  InitialCurrent=0  Capacitance=1e-6  Setx0=off  InitialVoltage=0  Measurements=None
  Conn1 : PMIOPort  Side=Left
  Conn2 : PMIOPort  Port=2  Side=Right
  Conn3 : PMIOPort  Port=3  Side=Left
  Conn4 : PMIOPort  Port=4  Side=Right
  Conn5 : PMIOPort  Port=5  Side=Left
  Conn6 : PMIOPort  Port=6  Side=Right
  Conn7 : PMIOPort  Port=7  Side=Left
  Conn8 : PMIOPort  Port=8  Side=Right
  Conn9 : PMIOPort  Port=9  Side=Left
  Conn10 : PMIOPort  Port=10  Side=Right
  Conn11 : PMIOPort  Port=11  Side=Left
  Conn12 : PMIOPort  Port=12  Side=Right
  Conn13 : PMIOPort  Port=13  Side=Left
  Conn14 : PMIOPort  Port=14  Side=Right
  Conn15 : PMIOPort  Port=15  Side=Left
  Conn16 : PMIOPort  Port=16  Side=Right
  Conn17 : PMIOPort  Port=17  Side=Left
  Conn18 : PMIOPort  Port=18  Side=Right
  connections:
  Series RLC Branch2/RConn1 -- Conn6/RConn1
  Series RLC Branch6/LConn1 -- Conn13/RConn1
  Series RLC Branch8/RConn1 -- Conn16/RConn1
  Series RLC Branch9/RConn1 -- Conn18/RConn1
  Series RLC Branch6/RConn1 -- Conn14/RConn1
  Series RLC Branch8/LConn1 -- Conn15/RConn1
  Series RLC Branch9/LConn1 -- Conn17/RConn1
  Series RLC Branch5/RConn1 -- Conn12/RConn1
  Series RLC Branch1/RConn1 -- Conn4/RConn1
  Series RLC Branch4/RConn1 -- Conn10/RConn1
  Series RLC Branch5/LConn1 -- Conn11/RConn1
  Series RLC Branch4/LConn1 -- Conn9/RConn1
  Series RLC Branch2/LConn1 -- Conn5/RConn1
  Series RLC Branch1/LConn1 -- Conn3/RConn1
  Series RLC Branch7/RConn1 -- Conn2/RConn1
  Series RLC Branch7/LConn1 -- Conn1/RConn1
  Series RLC Branch3/LConn1 -- Conn7/RConn1
  Series RLC Branch3/RConn1 -- Conn8/RConn1

== system model_sim_CHBjt7/Subsystem5 ==
  Series RLC Branch{1..9} (9 alike) : spsSeriesRLCBranchLib/Series RLC Branch  LConnTagsString=__new0  RConnTagsString=__new0  BranchType=L  Resistance=R*1.5  Inductance=L_in  SetiL0=off  InitialCurrent=0  Capacitance=1e-6  Setx0=off  InitialVoltage=0  Measurements=None
  Conn1 : PMIOPort  Side=Left
  Conn2 : PMIOPort  Port=2  Side=Right
  Conn3 : PMIOPort  Port=3  Side=Left
  Conn4 : PMIOPort  Port=4  Side=Right
  Conn5 : PMIOPort  Port=5  Side=Left
  Conn6 : PMIOPort  Port=6  Side=Right
  Conn7 : PMIOPort  Port=7  Side=Left
  Conn8 : PMIOPort  Port=8  Side=Right
  Conn9 : PMIOPort  Port=9  Side=Left
  Conn10 : PMIOPort  Port=10  Side=Right
  Conn11 : PMIOPort  Port=11  Side=Left
  Conn12 : PMIOPort  Port=12  Side=Right
  Conn13 : PMIOPort  Port=13  Side=Left
  Conn14 : PMIOPort  Port=14  Side=Right
  Conn15 : PMIOPort  Port=15  Side=Left
  Conn16 : PMIOPort  Port=16  Side=Right
  Conn17 : PMIOPort  Port=17  Side=Left
  Conn18 : PMIOPort  Port=18  Side=Right
  connections:
  Series RLC Branch3/RConn1 -- Conn8/RConn1
  Series RLC Branch3/LConn1 -- Conn7/RConn1
  Series RLC Branch7/LConn1 -- Conn1/RConn1
  Series RLC Branch7/RConn1 -- Conn2/RConn1
  Series RLC Branch1/LConn1 -- Conn3/RConn1
  Series RLC Branch2/LConn1 -- Conn5/RConn1
  Series RLC Branch4/LConn1 -- Conn9/RConn1
  Series RLC Branch5/LConn1 -- Conn11/RConn1
  Series RLC Branch4/RConn1 -- Conn10/RConn1
  Series RLC Branch1/RConn1 -- Conn4/RConn1
  Series RLC Branch5/RConn1 -- Conn12/RConn1
  Series RLC Branch9/LConn1 -- Conn17/RConn1
  Series RLC Branch8/LConn1 -- Conn15/RConn1
  Series RLC Branch6/RConn1 -- Conn14/RConn1
  Series RLC Branch9/RConn1 -- Conn18/RConn1
  Series RLC Branch8/RConn1 -- Conn16/RConn1
  Series RLC Branch6/LConn1 -- Conn13/RConn1
  Series RLC Branch2/RConn1 -- Conn6/RConn1

== system model_sim_CHBjt7/Subsystem6 ==
  Multi-Winding Transformer10 : spsMultiWindingTransformerLib/Multi-Winding Transformer  LeftWindings=1  RightWindings=5  TappedWindings=no taps  NumberOfTaps=2  SetSaturation=off  Hysteresis=off  DataFile='hysteresis.mat'  Measurements=None  UNITS=pu  NominalPower=[P0 fn]  NominalVoltages="[ Source_Amp   (1-sin(10/180*pi)/sin(50/180*pi))*2*sin(50/180*pi)*Ul_in sin(10/180*pi)/sin(50/180*pi)*2*sin(50/180*pi)*Ul_in  Ul_in (1-sin(10/180*pi)/sin(50/180*pi))*2*sin(50/180*pi)*Ul_in sin(10/180*pi)/sin(50/180*pi)*2*sin(50/180*pi)*Ul_in]"  WindingResistances="[ 0.005   0.005 0.005 0.005  0.005  0.005]"  WindingInductances="[ L_ori*5  L_sec L_sec L_sec L_sec L_sec]/5"  Rm=50  Lm=50  Saturation=[ 0,0 ; 0.0024,1.2 ; 1.0,1.52 ]  SpecifyInitialFlux=off  InitialFlux=0  BreakLoop=off  DiscreteSolver=Trapezoidal iterative  DataType=off  TransfoNumber=1
      settings: LibrarySourceBlock=|
      | sps_lib/Power Grid Elements/Multi-Winding
      | Transformer
  Multi-Winding Transformer11 : spsMultiWindingTransformerLib/Multi-Winding Transformer  LeftWindings=1  RightWindings=5  TappedWindings=no taps  NumberOfTaps=2  SetSaturation=off  Hysteresis=off  DataFile='hysteresis.mat'  Measurements=None  UNITS=pu  NominalPower=[P0 fn]  NominalVoltages="[ Source_Amp   (1-sin(10/180*pi)/sin(50/180*pi))*2*sin(50/180*pi)*Ul_in sin(10/180*pi)/sin(50/180*pi)*2*sin(50/180*pi)*Ul_in  Ul_in (1-sin(10/180*pi)/sin(50/180*pi))*2*sin(50/180*pi)*Ul_in sin(10/180*pi)/sin(50/180*pi)*2*sin(50/180*pi)*Ul_in]"  WindingResistances="[ 0.005   0.005 0.005 0.005  0.005  0.005]"  WindingInductances="[ L_ori*5  L_sec L_sec L_sec L_sec L_sec]/5"  Rm=50  Lm=50  Saturation=[ 0,0 ; 0.0024,1.2 ; 1.0,1.52 ]  SpecifyInitialFlux=off  InitialFlux=0  BreakLoop=off  DiscreteSolver=Trapezoidal iterative  DataType=off  TransfoNumber=1
      settings: LibrarySourceBlock=|
      | sps_lib/Power Grid Elements/Multi-Winding
      | Transformer
  Multi-Winding Transformer9 : spsMultiWindingTransformerLib/Multi-Winding Transformer  LeftWindings=1  RightWindings=5  TappedWindings=no taps  NumberOfTaps=2  SetSaturation=off  Hysteresis=off  DataFile='hysteresis.mat'  Measurements=None  UNITS=pu  NominalPower=[P0 fn]  NominalVoltages="[ Source_Amp (1-sin(10/180*pi)/sin(50/180*pi))*2*sin(50/180*pi)*Ul_in sin(10/180*pi)/sin(50/180*pi)*2*sin(50/180*pi)*Ul_in  Ul_in (1-sin(10/180*pi)/sin(50/180*pi))*2*sin(50/180*pi)*Ul_in sin(10/180*pi)/sin(50/180*pi)*2*sin(50/180*pi)*Ul_in]"  WindingResistances="[ 0.005   0.005 0.005 0.005  0.005  0.005]"  WindingInductances="[ L_ori*5  L_sec L_sec L_sec L_sec L_sec]/5"  Rm=50  Lm=50  Saturation=[ 0,0 ; 0.0024,1.2 ; 1.0,1.52 ]  SpecifyInitialFlux=off  InitialFlux=0  BreakLoop=off  DiscreteSolver=Trapezoidal iterative  DataType=off  TransfoNumber=1
      settings: LibrarySourceBlock=|
      | sps_lib/Power Grid Elements/Multi-Winding
      | Transformer
  1+ : PMIOPort  Side=Left
  1+1 : PMIOPort  Port=2  Side=Left
  1+2 : PMIOPort  Port=3  Side=Left
  -20a : PMIOPort  Port=4  Side=Right
  -20b : PMIOPort  Port=5  Side=Right
  -20c : PMIOPort  Port=6  Side=Right
  0a : PMIOPort  Port=7  Side=Right
  0b : PMIOPort  Port=8  Side=Right
  0c : PMIOPort  Port=9  Side=Right
  +20a : PMIOPort  Port=10  Side=Right
  +20b : PMIOPort  Port=11  Side=Right
  +20c : PMIOPort  Port=12  Side=Right
  connections:
  Multi-Winding Transformer10/RConn9 -- +20b/RConn1
  Multi-Winding Transformer10/RConn5 -- 0b/RConn1
  Multi-Winding Transformer9/LConn1 -- 1+/RConn1
  Multi-Winding Transformer11/RConn9 -- +20c/RConn1
  +20a/RConn1 -- Multi-Winding Transformer9/RConn9
  Multi-Winding Transformer10/LConn1 -- 1+1/RConn1
  Multi-Winding Transformer9/RConn5 -- 0a/RConn1
  -20a/RConn1 -- Multi-Winding Transformer9/RConn3
  Multi-Winding Transformer11/RConn5 -- 0c/RConn1
  Multi-Winding Transformer11/LConn1 -- 1+2/RConn1
  Multi-Winding Transformer11/RConn3 -- -20c/RConn1
  Multi-Winding Transformer11/RConn2 -- Multi-Winding Transformer10/RConn4 -- Multi-Winding Transformer10/RConn1
  Multi-Winding Transformer10/RConn3 -- -20b/RConn1
  Multi-Winding Transformer11/RConn8 -- Multi-Winding Transformer9/RConn7 -- Multi-Winding Transformer9/RConn10
  Multi-Winding Transformer11/RConn4 -- Multi-Winding Transformer9/RConn2 -- Multi-Winding Transformer11/RConn1
  Multi-Winding Transformer10/RConn10 -- Multi-Winding Transformer9/RConn8 -- Multi-Winding Transformer10/RConn7
  Multi-Winding Transformer11/RConn6 -- Multi-Winding Transformer9/RConn6 -- Multi-Winding Transformer10/RConn6
  Multi-Winding Transformer10/RConn2 -- Multi-Winding Transformer9/RConn4 -- Multi-Winding Transformer9/RConn1
  Multi-Winding Transformer11/RConn10 -- Multi-Winding Transformer10/RConn8 -- Multi-Winding Transformer11/RConn7
  Multi-Winding Transformer11/LConn2 -- Multi-Winding Transformer9/LConn2 -- Multi-Winding Transformer10/LConn2

== system model_sim_CHBjt7/Subsystem7 ==
  Multi-Winding Transformer10 : spsMultiWindingTransformerLib/Multi-Winding Transformer  LeftWindings=1  RightWindings=5  TappedWindings=no taps  NumberOfTaps=2  SetSaturation=off  Hysteresis=off  DataFile='hysteresis.mat'  Measurements=None  UNITS=pu  NominalPower=[P0 fn]  NominalVoltages="[ Source_Amp   (1-sin(10/180*pi)/sin(50/180*pi))*2*sin(50/180*pi)*Ul_in sin(10/180*pi)/sin(50/180*pi)*2*sin(50/180*pi)*Ul_in  Ul_in (1-sin(10/180*pi)/sin(50/180*pi))*2*sin(50/180*pi)*Ul_in sin(10/180*pi)/sin(50/180*pi)*2*sin(50/180*pi)*Ul_in]"  WindingResistances="[ 0.005   0.005 0.005 0.005  0.005  0.005]"  WindingInductances="[ L_ori*5  L_sec L_sec L_sec L_sec L_sec]/5"  Rm=50  Lm=50  Saturation=[ 0,0 ; 0.0024,1.2 ; 1.0,1.52 ]  SpecifyInitialFlux=off  InitialFlux=0  BreakLoop=off  DiscreteSolver=Trapezoidal iterative  DataType=off  TransfoNumber=1
      settings: LibrarySourceBlock=|
      | sps_lib/Power Grid Elements/Multi-Winding
      | Transformer
  Multi-Winding Transformer11 : spsMultiWindingTransformerLib/Multi-Winding Transformer  LeftWindings=1  RightWindings=5  TappedWindings=no taps  NumberOfTaps=2  SetSaturation=off  Hysteresis=off  DataFile='hysteresis.mat'  Measurements=None  UNITS=pu  NominalPower=[P0 fn]  NominalVoltages="[ Source_Amp   (1-sin(10/180*pi)/sin(50/180*pi))*2*sin(50/180*pi)*Ul_in sin(10/180*pi)/sin(50/180*pi)*2*sin(50/180*pi)*Ul_in  Ul_in (1-sin(10/180*pi)/sin(50/180*pi))*2*sin(50/180*pi)*Ul_in sin(10/180*pi)/sin(50/180*pi)*2*sin(50/180*pi)*Ul_in]"  WindingResistances="[ 0.005   0.005 0.005 0.005  0.005  0.005]"  WindingInductances="[ L_ori*5  L_sec L_sec L_sec L_sec L_sec]/5"  Rm=50  Lm=50  Saturation=[ 0,0 ; 0.0024,1.2 ; 1.0,1.52 ]  SpecifyInitialFlux=off  InitialFlux=0  BreakLoop=off  DiscreteSolver=Trapezoidal iterative  DataType=off  TransfoNumber=1
      settings: LibrarySourceBlock=|
      | sps_lib/Power Grid Elements/Multi-Winding
      | Transformer
  Multi-Winding Transformer9 : spsMultiWindingTransformerLib/Multi-Winding Transformer  LeftWindings=1  RightWindings=5  TappedWindings=no taps  NumberOfTaps=2  SetSaturation=off  Hysteresis=off  DataFile='hysteresis.mat'  Measurements=None  UNITS=pu  NominalPower=[P0 fn]  NominalVoltages="[ Source_Amp (1-sin(10/180*pi)/sin(50/180*pi))*2*sin(50/180*pi)*Ul_in sin(10/180*pi)/sin(50/180*pi)*2*sin(50/180*pi)*Ul_in  Ul_in (1-sin(10/180*pi)/sin(50/180*pi))*2*sin(50/180*pi)*Ul_in sin(10/180*pi)/sin(50/180*pi)*2*sin(50/180*pi)*Ul_in]"  WindingResistances="[ 0.005   0.005 0.005 0.005  0.005  0.005]"  WindingInductances="[ L_ori*5  L_sec L_sec L_sec L_sec L_sec]/5"  Rm=50  Lm=50  Saturation=[ 0,0 ; 0.0024,1.2 ; 1.0,1.52 ]  SpecifyInitialFlux=off  InitialFlux=0  BreakLoop=off  DiscreteSolver=Trapezoidal iterative  DataType=off  TransfoNumber=1
      settings: LibrarySourceBlock=|
      | sps_lib/Power Grid Elements/Multi-Winding
      | Transformer
  1+ : PMIOPort  Side=Left
  1+1 : PMIOPort  Port=2  Side=Left
  1+2 : PMIOPort  Port=3  Side=Left
  -20a : PMIOPort  Port=4  Side=Right
  -20b : PMIOPort  Port=5  Side=Right
  -20c : PMIOPort  Port=6  Side=Right
  0a : PMIOPort  Port=7  Side=Right
  0b : PMIOPort  Port=8  Side=Right
  0c : PMIOPort  Port=9  Side=Right
  +20a : PMIOPort  Port=10  Side=Right
  +20b : PMIOPort  Port=11  Side=Right
  +20c : PMIOPort  Port=12  Side=Right
  connections:
  Multi-Winding Transformer10/LConn2 -- Multi-Winding Transformer9/LConn2 -- Multi-Winding Transformer11/LConn2
  Multi-Winding Transformer11/RConn7 -- Multi-Winding Transformer10/RConn8 -- Multi-Winding Transformer11/RConn10
  Multi-Winding Transformer9/RConn1 -- Multi-Winding Transformer9/RConn4 -- Multi-Winding Transformer10/RConn2
  Multi-Winding Transformer10/RConn6 -- Multi-Winding Transformer9/RConn6 -- Multi-Winding Transformer11/RConn6
  Multi-Winding Transformer10/RConn7 -- Multi-Winding Transformer9/RConn8 -- Multi-Winding Transformer10/RConn10
  Multi-Winding Transformer11/RConn1 -- Multi-Winding Transformer9/RConn2 -- Multi-Winding Transformer11/RConn4
  Multi-Winding Transformer9/RConn10 -- Multi-Winding Transformer9/RConn7 -- Multi-Winding Transformer11/RConn8
  Multi-Winding Transformer10/RConn3 -- -20b/RConn1
  Multi-Winding Transformer10/RConn1 -- Multi-Winding Transformer10/RConn4 -- Multi-Winding Transformer11/RConn2
  Multi-Winding Transformer11/RConn3 -- -20c/RConn1
  Multi-Winding Transformer11/LConn1 -- 1+2/RConn1
  Multi-Winding Transformer11/RConn5 -- 0c/RConn1
  -20a/RConn1 -- Multi-Winding Transformer9/RConn3
  Multi-Winding Transformer9/RConn5 -- 0a/RConn1
  Multi-Winding Transformer10/LConn1 -- 1+1/RConn1
  +20a/RConn1 -- Multi-Winding Transformer9/RConn9
  Multi-Winding Transformer11/RConn9 -- +20c/RConn1
  Multi-Winding Transformer9/LConn1 -- 1+/RConn1
  Multi-Winding Transformer10/RConn5 -- 0b/RConn1
  Multi-Winding Transformer10/RConn9 -- +20b/RConn1

== system model_sim_CHBjt7/Subsystem8 ==
  Multi-Winding Transformer10 : spsMultiWindingTransformerLib/Multi-Winding Transformer  LeftWindings=1  RightWindings=5  TappedWindings=no taps  NumberOfTaps=2  SetSaturation=off  Hysteresis=off  DataFile='hysteresis.mat'  Measurements=None  UNITS=pu  NominalPower=[P0 fn]  NominalVoltages="[ Source_Amp   (1-sin(10/180*pi)/sin(50/180*pi))*2*sin(50/180*pi)*Ul_in sin(10/180*pi)/sin(50/180*pi)*2*sin(50/180*pi)*Ul_in  Ul_in (1-sin(10/180*pi)/sin(50/180*pi))*2*sin(50/180*pi)*Ul_in sin(10/180*pi)/sin(50/180*pi)*2*sin(50/180*pi)*Ul_in]"  WindingResistances="[ 0.005   0.005 0.005 0.005  0.005  0.005]"  WindingInductances="[ L_ori*5  L_sec L_sec L_sec L_sec L_sec]/5"  Rm=50  Lm=50  Saturation=[ 0,0 ; 0.0024,1.2 ; 1.0,1.52 ]  SpecifyInitialFlux=off  InitialFlux=0  BreakLoop=off  DiscreteSolver=Trapezoidal iterative  DataType=off  TransfoNumber=1
      settings: LibrarySourceBlock=|
      | sps_lib/Power Grid Elements/Multi-Winding
      | Transformer
  Multi-Winding Transformer11 : spsMultiWindingTransformerLib/Multi-Winding Transformer  LeftWindings=1  RightWindings=5  TappedWindings=no taps  NumberOfTaps=2  SetSaturation=off  Hysteresis=off  DataFile='hysteresis.mat'  Measurements=None  UNITS=pu  NominalPower=[P0 fn]  NominalVoltages="[ Source_Amp   (1-sin(10/180*pi)/sin(50/180*pi))*2*sin(50/180*pi)*Ul_in sin(10/180*pi)/sin(50/180*pi)*2*sin(50/180*pi)*Ul_in  Ul_in (1-sin(10/180*pi)/sin(50/180*pi))*2*sin(50/180*pi)*Ul_in sin(10/180*pi)/sin(50/180*pi)*2*sin(50/180*pi)*Ul_in]"  WindingResistances="[ 0.005   0.005 0.005 0.005  0.005  0.005]"  WindingInductances="[ L_ori*5  L_sec L_sec L_sec L_sec L_sec]/5"  Rm=50  Lm=50  Saturation=[ 0,0 ; 0.0024,1.2 ; 1.0,1.52 ]  SpecifyInitialFlux=off  InitialFlux=0  BreakLoop=off  DiscreteSolver=Trapezoidal iterative  DataType=off  TransfoNumber=1
      settings: LibrarySourceBlock=|
      | sps_lib/Power Grid Elements/Multi-Winding
      | Transformer
  Multi-Winding Transformer9 : spsMultiWindingTransformerLib/Multi-Winding Transformer  LeftWindings=1  RightWindings=5  TappedWindings=no taps  NumberOfTaps=2  SetSaturation=off  Hysteresis=off  DataFile='hysteresis.mat'  Measurements=None  UNITS=pu  NominalPower=[P0 fn]  NominalVoltages="[ Source_Amp (1-sin(10/180*pi)/sin(50/180*pi))*2*sin(50/180*pi)*Ul_in sin(10/180*pi)/sin(50/180*pi)*2*sin(50/180*pi)*Ul_in  Ul_in (1-sin(10/180*pi)/sin(50/180*pi))*2*sin(50/180*pi)*Ul_in sin(10/180*pi)/sin(50/180*pi)*2*sin(50/180*pi)*Ul_in]"  WindingResistances="[ 0.005   0.005 0.005 0.005  0.005  0.005]"  WindingInductances="[ L_ori*5  L_sec L_sec L_sec L_sec L_sec]/5"  Rm=50  Lm=50  Saturation=[ 0,0 ; 0.0024,1.2 ; 1.0,1.52 ]  SpecifyInitialFlux=off  InitialFlux=0  BreakLoop=off  DiscreteSolver=Trapezoidal iterative  DataType=off  TransfoNumber=1
      settings: LibrarySourceBlock=|
      | sps_lib/Power Grid Elements/Multi-Winding
      | Transformer
  1+ : PMIOPort  Side=Left
  1+1 : PMIOPort  Port=2  Side=Left
  1+2 : PMIOPort  Port=3  Side=Left
  -20a : PMIOPort  Port=4  Side=Right
  -20b : PMIOPort  Port=5  Side=Right
  -20c : PMIOPort  Port=6  Side=Right
  0a : PMIOPort  Port=7  Side=Right
  0b : PMIOPort  Port=8  Side=Right
  0c : PMIOPort  Port=9  Side=Right
  +20a : PMIOPort  Port=10  Side=Right
  +20b : PMIOPort  Port=11  Side=Right
  +20c : PMIOPort  Port=12  Side=Right
  connections:
  Multi-Winding Transformer10/LConn2 -- Multi-Winding Transformer9/LConn2 -- Multi-Winding Transformer11/LConn2
  Multi-Winding Transformer11/RConn7 -- Multi-Winding Transformer10/RConn8 -- Multi-Winding Transformer11/RConn10
  Multi-Winding Transformer9/RConn1 -- Multi-Winding Transformer9/RConn4 -- Multi-Winding Transformer10/RConn2
  Multi-Winding Transformer10/RConn6 -- Multi-Winding Transformer9/RConn6 -- Multi-Winding Transformer11/RConn6
  Multi-Winding Transformer10/RConn7 -- Multi-Winding Transformer9/RConn8 -- Multi-Winding Transformer10/RConn10
  Multi-Winding Transformer11/RConn1 -- Multi-Winding Transformer9/RConn2 -- Multi-Winding Transformer11/RConn4
  Multi-Winding Transformer9/RConn10 -- Multi-Winding Transformer9/RConn7 -- Multi-Winding Transformer11/RConn8
  Multi-Winding Transformer10/RConn3 -- -20b/RConn1
  Multi-Winding Transformer10/RConn1 -- Multi-Winding Transformer10/RConn4 -- Multi-Winding Transformer11/RConn2
  Multi-Winding Transformer11/RConn3 -- -20c/RConn1
  Multi-Winding Transformer11/LConn1 -- 1+2/RConn1
  Multi-Winding Transformer11/RConn5 -- 0c/RConn1
  -20a/RConn1 -- Multi-Winding Transformer9/RConn3
  Multi-Winding Transformer9/RConn5 -- 0a/RConn1
  Multi-Winding Transformer10/LConn1 -- 1+1/RConn1
  +20a/RConn1 -- Multi-Winding Transformer9/RConn9
  Multi-Winding Transformer11/RConn9 -- +20c/RConn1
  Multi-Winding Transformer9/LConn1 -- 1+/RConn1
  Multi-Winding Transformer10/RConn5 -- 0b/RConn1
  Multi-Winding Transformer10/RConn9 -- +20b/RConn1
